simulink model "Hinf_simulation1"  (R2023a)
settings: Solver=VariableStepAuto  StartTime=0.0  StopTime=10.0  RelTol=1e-3
values from neighbouring files (symbols this model uses):
  C = [1 0 0 0; 0 1 0 0]    [Hinf_1DOF.m]    (also in Hinf_2DOFinit.m; Hinf_U_init.m; Hinf_WU_init.m; Hinf_init.m)
  dtheta_0 = 0    [Hinf_1DOF.m]    (also in Hinf_2DOFinit.m; Hinf_U_init.m; Hinf_WU_init.m; Hinf_init.m)
  dz_0 = 0    [Hinf_1DOF.m]    (also in Hinf_2DOFinit.m; Hinf_U_init.m; Hinf_WU_init.m; Hinf_init.m)
  fa_w = 0    [Hinf_1DOF.m]    (also in Hinf_2DOFinit.m; Hinf_U_init.m; Hinf_WU_init.m; Hinf_init.m)
  fm_w = s_param.g*s_param.m    [Hinf_1DOF.m]    (also in Hinf_2DOFinit.m; Hinf_U_init.m; Hinf_WU_init.m; Hinf_init.m)
  Km1 = 1.1    [Hinf_1DOF.m]    (also in Hinf_2DOFinit.m; Hinf_U_init.m; Hinf_WU_init.m; Hinf_init.m)
  Km2 = 1.1    [Hinf_1DOF.m]    (also in Hinf_2DOFinit.m; Hinf_U_init.m; Hinf_WU_init.m; Hinf_init.m)
  out_rate = 0.001    [Hinf_1DOF.m]    (also in Hinf_2DOFinit.m; Hinf_U_init.m; Hinf_WU_init.m; Hinf_init.m)
  T1 = 0.05    [Hinf_1DOF.m]    (also in Hinf_2DOFinit.m; Hinf_U_init.m; Hinf_WU_init.m; Hinf_init.m)
  T2 = 0.15    [Hinf_1DOF.m]    (also in Hinf_2DOFinit.m; Hinf_U_init.m; Hinf_WU_init.m; Hinf_init.m)
  theta_0_real = theta_0 + std_dev.theta_0*randn(1,1)    [Hinf_1DOF.m]    (also in Hinf_2DOFinit.m = theta_0+std_dev.theta_0*randn(1,1); Hinf_U_init.m = theta_0+std_dev.theta_0*randn(1,1); Hinf_WU_init.m = theta_0+std_dev.theta_0*randn(1,1); Hinf_init.m = theta_0+std_dev.theta_0*randn(1,1))
  Tm1 = 1    [Hinf_1DOF.m]    (also in Hinf_2DOFinit.m; Hinf_U_init.m; Hinf_WU_init.m; Hinf_init.m)
  Tm2 = 1    [Hinf_1DOF.m]    (also in Hinf_2DOFinit.m; Hinf_U_init.m; Hinf_WU_init.m; Hinf_init.m)
  z_0_real = z_0 + std_dev.z_0*randn(1,1)    [Hinf_1DOF.m]    (also in Hinf_2DOFinit.m = z_0+std_dev.z_0*randn(1,1); Hinf_U_init.m = z_0+std_dev.z_0*randn(1,1); Hinf_WU_init.m = z_0+std_dev.z_0*randn(1,1); Hinf_init.m = z_0+std_dev.z_0*randn(1,1))
undefined symbols (not defined in the file or in its folder): std_dev
libraries: simulink x2
settings Model: Creator=franc  LastModifiedBy=franc

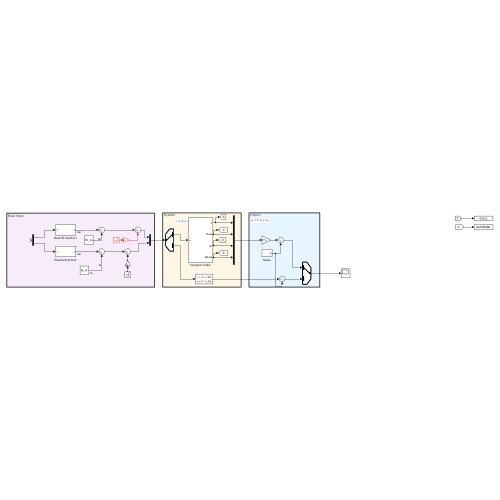
[thumbnail: Simulink's stored preview of the top-level diagram]
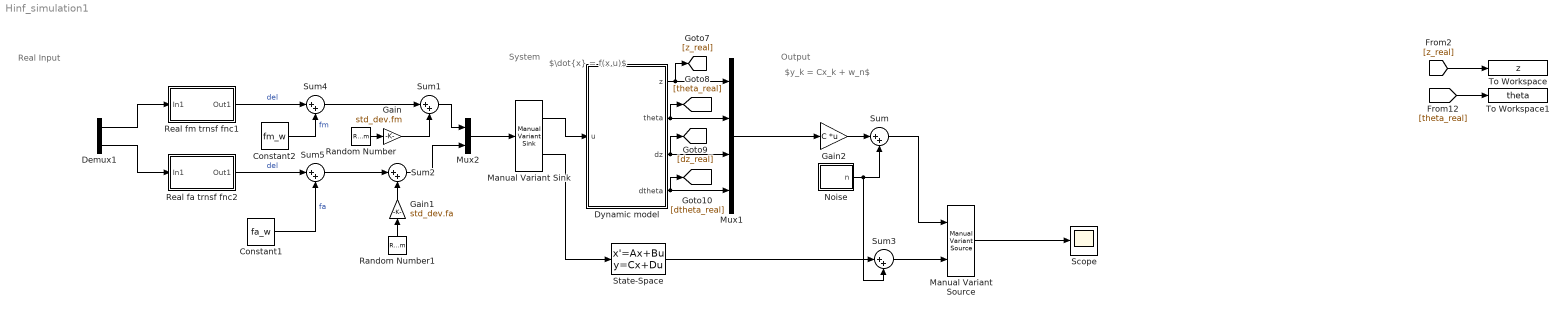
== system Hinf_simulation1 ==
  note: System
  note: $y_k = Cx_k + w_n$
  note: $\dot{x} = f(x,u)$
  note: Output
  note: Real Input
  Constant1 : Constant  Value=fa_w
  Constant2 : Constant  Value=fm_w
  Demux1 : Demux  Outputs=2
  Dynamic model : Subsystem
  Gain : Gain  Gain=std_dev.fm
  Gain1 : Gain  Gain=std_dev.fa
  Gain2 : Gain  Gain=C  Multiplication=Matrix(K*u)
  Manual Variant Sink : simulink/Signal Routing/Manual Variant Sink  NumChoices=2  LabelModeActiveChoice=V_1
  Manual Variant Source : simulink/Signal Routing/Manual Variant Source  NumChoices=2  LabelModeActiveChoice=V_1
  Mux1 : Mux
  Mux2 : Mux  Inputs=2
  Noise : Subsystem
  Random Number : RandomNumber  SampleTime=out_rate
  Random Number1 : RandomNumber  SampleTime=out_rate
  Real fa trnsf fnc2 : Subsystem
  Real fm trnsf fnc1 : Subsystem
  Scope : Scope
  State-Space : StateSpace  InitialCondition=0
  Sum{,1..5} (6 alike) : Sum  Inputs=|++
  To Workspace : ToWorkspace  VariableName=z  SaveFormat=Timeseries  SampleTime=-1
  To Workspace1 : ToWorkspace  VariableName=theta  SaveFormat=Timeseries  SampleTime=-1
  wires:
  Real fm trnsf fnc1/1(Out1) -> Sum4/1  "del"
  [theta_real] -> To Workspace1/1
  [z_real] -> To Workspace/1
  State-Space/1 -> Sum3/1
  Manual Variant Sink/2 -> State-Space/1
  Mux2/1 -> Manual Variant Sink/1
  Constant1/1 -> Sum5/2  "fa"
  Gain/1 -> Sum1/2
  Sum2/1 -> Mux2/2
  Sum4/1 -> Sum1/1
  Random Number/1 -> Gain/1
  Random Number1/1 -> Gain1/1
  Gain1/1 -> Sum2/2
  Dynamic model/1(z) -> [z_real], Mux1/1
  Sum5/1 -> Sum2/1
  Dynamic model/4(dtheta) -> Mux1/4, [dtheta_real]
  Sum1/1 -> Mux2/1
  Constant2/1 -> Sum4/2  "fm"
  Demux1/1 -> Real fm trnsf fnc1/1(In1)
  Dynamic model/3(dz) -> Mux1/3, [dz_real]
  Real fa trnsf fnc2/1(Out1) -> Sum5/1  "del"
  Mux1/1 -> Gain2/1
  Manual Variant Sink/1 -> Dynamic model/1(u)
  Dynamic model/2(theta) -> Mux1/2, [theta_real]
  Demux1/2 -> Real fa trnsf fnc2/1(In1)
  Manual Variant Source/1 -> Scope/1
  Gain2/1 -> Sum/1
  Sum/1 -> Manual Variant Source/1
  Noise/1(n) -> Sum/2, Sum3/2
  Sum3/1 -> Manual Variant Source/2

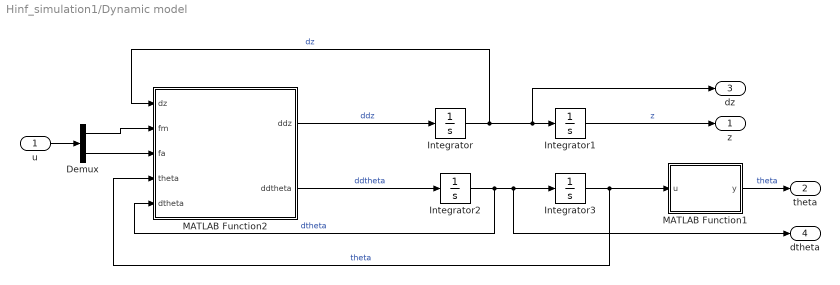
== system Hinf_simulation1/Dynamic model ==
  u : Inport
  Demux : Demux  Outputs=2
  Integrator : Integrator  InitialCondition=dz_0
  Integrator1 : Integrator  InitialCondition=z_0_real
  Integrator2 : Integrator  InitialCondition=dtheta_0
  Integrator3 : Integrator  InitialCondition=theta_0_real
  MATLAB Function1 : MATLAB Function  TreatAsAtomicUnit=on
  MATLAB Function2 : MATLAB Function  TreatAsAtomicUnit=on
  z : Outport
  theta : Outport  Port=2
  dz : Outport  Port=3
  dtheta : Outport  Port=4
  wires:
  Integrator3/1 -> MATLAB Function2/4(theta), MATLAB Function1/1(u)  "theta"
  Integrator2/1 -> dtheta/1, Integrator3/1, MATLAB Function2/5(dtheta)  "dtheta"
  MATLAB Function1/1(y) -> theta/1  "theta"
  Integrator1/1 -> z/1  "z"
  MATLAB Function2/2(ddtheta) -> Integrator2/1  "ddtheta"
  MATLAB Function2/1(ddz) -> Integrator/1  "ddz"
  Integrator/1 -> dz/1, Integrator1/1, MATLAB Function2/1(dz)  "dz"
  u/1 -> Demux/1
  Demux/2 -> MATLAB Function2/3(fa)
  Demux/1 -> MATLAB Function2/2(fm)

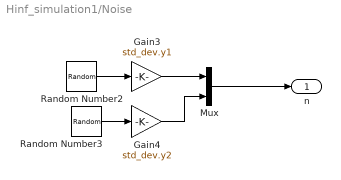
== system Hinf_simulation1/Noise ==
  Gain3 : Gain  Gain=std_dev.y1
  Gain4 : Gain  Gain=std_dev.y2
  Mux : Mux  Inputs=2
  Random Number2 : RandomNumber  SampleTime=0.1
  Random Number3 : RandomNumber  SampleTime=0.1
  n : Outport
  wires:
  Random Number2/1 -> Gain3/1
  Random Number3/1 -> Gain4/1
  Gain4/1 -> Mux/2
  Mux/1 -> n/1
  Gain3/1 -> Mux/1

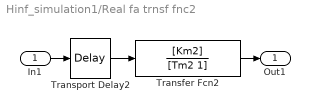
== system Hinf_simulation1/Real fa trnsf fnc2 ==
  In1 : Inport
  Transfer Fcn2 : TransferFcn  Numerator=[Km2]  Denominator=[Tm2 1]
  Transport Delay2 : TransportDelay  DelayTime=T2
  Out1 : Outport
  wires:
  Transport Delay2/1 -> Transfer Fcn2/1
  Transfer Fcn2/1 -> Out1/1
  In1/1 -> Transport Delay2/1

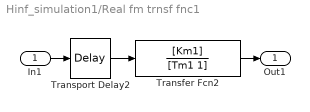
== system Hinf_simulation1/Real fm trnsf fnc1 ==
  In1 : Inport
  Transfer Fcn2 : TransferFcn  Numerator=[Km1]  Denominator=[Tm1 1]
  Transport Delay2 : TransportDelay  DelayTime=T1
  Out1 : Outport
  wires:
  In1/1 -> Transport Delay2/1
  Transfer Fcn2/1 -> Out1/1
  Transport Delay2/1 -> Transfer Fcn2/1

== matlab function Hinf_simulation1/Dynamic model/MATLAB Function2 ==
  data: dz input; fm input; fa input; ddz output; ddtheta output; theta input; dtheta input; s_param parameter
function [ddz, ddtheta] = fcn(dz, fm, fa, theta, dtheta, s_param)

% Rename params
J = s_param.J;     
m = s_param.m;     
b = s_param.b;      
beta = s_param.beta;    
g = s_param.g;     
l = s_param.l;   

%% Dynamic equations

ddz = -b/m * dz + fm/m * cos(theta) -g;
ddtheta = -beta/J * dtheta + 2 * l/J * fa;

end

== matlab function Hinf_simulation1/Dynamic model/MATLAB Function1 ==
  data: u input; y output
function y = fcn(u)

y = atan2(sin(u), cos(u));
end
